simulink model "generic_Truck_And_Trailer"  (R2025a)
settings: Solver=VariableStepAuto  StartTime=0.0  StopTime=350  FixedStep=0.01  MaxStep=0.001  RelTol=1e-3  EnableMultiTasking=on
libraries: TruckMaker4SL x250, simulink x1
(part 2 of 11)

== system generic_Truck_And_Trailer/TruckMaker/IPG Vehicle/CarAndTrailer ==
  Sync_In : Inport
  VhclCtrl.Steering : Inport  Port=2
  Vhcl.Wheel.In : Inport  Port=3
  Vhcl.Misc : Inport  Port=4
  CarAndTrailerUpd : Subsystem
  Forces : Subsystem
  Ground : Ground
  Kinematics : Subsystem
  Kinetics : Subsystem
  Steering : Subsystem
  Terminator : Terminator
  Terminator1 : Terminator
  Trailer : Subsystem
  Sync_Out : Outport  VectorParamsAs1DForOutWhenUnconnected=off
  Brake.IF.In : Outport  Port=2  VectorParamsAs1DForOutWhenUnconnected=off
  wires:
  Trailer/16(Vhcl.Wheel.RR4) -> CarAndTrailerUpd/16(Vhcl.Wheel.RR4)
  Trailer/15(Vhcl.Wheel.RL4) -> CarAndTrailerUpd/15(Vhcl.Wheel.RL4)
  Trailer/14(Vhcl.Wheel.RR3) -> CarAndTrailerUpd/14(Vhcl.Wheel.RR3)
  Trailer/13(Vhcl.Wheel.RL3) -> CarAndTrailerUpd/13(Vhcl.Wheel.RL3)
  Ground/1 -> CarAndTrailerUpd/18(Vhcl.Fr1A)
  Trailer/17(Car.Hitch.FrcTrq) -> CarAndTrailerUpd/17(Car.Hitch.FrcTrq)
  Trailer/12(Vhcl.Wheel.FR2) -> CarAndTrailerUpd/12(Vhcl.Wheel.FR2)
  Trailer/11(Vhcl.Wheel.FL2) -> CarAndTrailerUpd/11(Vhcl.Wheel.FL2)
  Trailer/10(Vhcl.Wheel.RR2) -> CarAndTrailerUpd/10(Vhcl.Wheel.RR2)
  Trailer/9(Vhcl.Wheel.RL2) -> CarAndTrailerUpd/9(Vhcl.Wheel.RL2)
  Trailer/8(Vhcl.Wheel.RR) -> CarAndTrailerUpd/8(Vhcl.Wheel.RR)
  Trailer/7(Vhcl.Wheel.RL) -> CarAndTrailerUpd/7(Vhcl.Wheel.RL)
  Trailer/6(Vhcl.Wheel.FR) -> CarAndTrailerUpd/6(Vhcl.Wheel.FR)
  Trailer/5(Vhcl.Wheel.FL) -> CarAndTrailerUpd/5(Vhcl.Wheel.FL)
  Trailer/4(Vhcl.PoI) -> CarAndTrailerUpd/4(Vhcl.PoI)
  Trailer/3(Vhcl.Motion) -> CarAndTrailerUpd/3(Vhcl.Motion)
  Trailer/2(Vhcl.Steering) -> CarAndTrailerUpd/2(Vhcl.Steering)
  Trailer/1(Sync_Out) -> CarAndTrailerUpd/1(Sync_In)
  CarAndTrailerUpd/2(Brake.IF.In) -> Brake.IF.In/1
  CarAndTrailerUpd/1(Sync_Out) -> Sync_Out/1
  Vhcl.Misc/1 -> Terminator1/1
  Vhcl.Wheel.In/1 -> Terminator/1
  Kinetics/6(WheelCarrier.Misc) -> Trailer/6(WheelCarrier.Misc)
  Kinetics/5(Car.Trq_T2W) -> Trailer/5(Car.Trq_T2W)
  Steering/2(Steer.IF) -> Kinematics/2(Steer.IF)
  Kinetics/4(Car.Fr1) -> Trailer/4(Car.Fr1)
  Kinetics/3(Car.Hitch) -> Trailer/3(Car.Hitch)
  Kinetics/2(Trailer.Load) -> Trailer/2(Trailer.Load)
  VhclCtrl.Steering/1 -> Steering/2(VhclCtrl.Steering)
  Sync_In/1 -> Steering/1(Sync_In)
  Steering/1(Sync_Out) -> Kinematics/1(Sync_In)
  Kinetics/1(Sync_Out) -> Trailer/1(Sync_In)
  Kinematics/5(lBuf) -> Forces/5(lBuf)
  Forces/4(Car.Load) -> Kinetics/4(Car.Load)
  Forces/2(Car.Virtual) -> Kinetics/2(Car.Virtual)
  Kinematics/2(lSpring) -> Forces/2(lSpring)
  Kinematics/3(vDamp) -> Forces/3(vDamp)
  Forces/3(Car.Aero) -> Kinetics/3(Car.Aero)
  Forces/1(Sync_Out) -> Kinetics/1(Sync_In)
  Kinematics/1(Sync_Out) -> Forces/1(Sync_In)
  Kinematics/4(lStabi) -> Forces/4(lStabi)
  Kinematics/6(tWheelCarrier_z) -> Forces/6(tWheelCarrier_z)

== system generic_Truck_And_Trailer/TruckMaker/IPG Vehicle/PowerTrain ==
  note: When replacing the entire powertrain,
      | be sure to disable the IPG powertrain model by using the powertrain
      | model 'Model Manager off' in the vehicle GUI.
  note: <Your model here>
  Sync_In : Inport
  Vhcl.Wheel.PT : Inport  Port=2
  VhclCtrl.PT : Inport  Port=3
  BusCreator : BusCreator  Inputs=99
  Demux : Demux  Outputs=99
      settings: DisplayOption=none
  Gain : Gain
  PowerTrain : S-Function  FunctionName=TM_Sfun  Parameters='PowerTrain'  SFunctionDeploymentMode=off  EnableBusSupport=off
  PowerTrainUpd : S-Function  FunctionName=TM_Sfun  Parameters='PowerTrainUpd'  SFunctionDeploymentMode=off  EnableBusSupport=off
  Sum : Sum  Inputs=|++
  Sync_Out : Outport  VectorParamsAs1DForOutWhenUnconnected=off
  WRR_Trq-drive : Outport  Port=2
  wires:
  Demux/97 -> BusCreator/97  "PT IF WRR4 Trq_Supp2WC"
  Demux/95 -> BusCreator/95  "PT IF WRR4 Trq_B2W"
  Demux/92 -> BusCreator/92  "PT IF WRL4 Trq_BrakeReg_max"
  Demux/88 -> BusCreator/88  "PT IF WRL4 Trq_B2W"
  Demux/89 -> BusCreator/89  "PT IF WRL4 Trq_Drive"
  Demux/86 -> BusCreator/86  "PT IF WRL4 rot"
  Demux/91 -> BusCreator/91  "PT IF WRL4 Trq_BrakeReg"
  Demux/84 -> BusCreator/84  "PT IF WRR3 Trq_BrakeReg"
  Demux/83 -> BusCreator/83  "PT IF WRR3 Trq_Supp2WC"
  Demux/82 -> BusCreator/82  "PT IF WRR3 Trq_Drive"
  Demux/78 -> BusCreator/78  "PT IF WRL3 Trq_BrakeReg_max"
  Demux/87 -> BusCreator/87  "PT IF WRL4 rotv"
  Demux/77 -> BusCreator/77  "PT IF WRL3 Trq_BrakeReg"
  Demux/75 -> BusCreator/75  "PT IF WRL3 Trq_Drive"
  Demux/73 -> BusCreator/73  "PT IF WRL3 rotv"
  Demux/72 -> BusCreator/72  "PT IF WRL3 rot"
  Demux/71 -> BusCreator/71  "PT IF WFR2 Trq_BrakeReg_max"
  Demux/70 -> BusCreator/70  "PT IF WFR2 Trq_BrakeReg"
  Demux/67 -> BusCreator/67  "PT IF WFR2 Trq_B2W"
  Demux/66 -> BusCreator/66  "PT IF WFR2 rotv"
  Demux/80 -> BusCreator/80  "PT IF WRR3 rotv"
  Demux/65 -> BusCreator/65  "PT IF WFR2 rot"
  Demux/76 -> BusCreator/76  "PT IF WRL3 Trq_Supp2WC"
  Demux/63 -> BusCreator/63  "PT IF WFL2 Trq_BrakeReg"
  Demux/74 -> BusCreator/74  "PT IF WRL3 Trq_B2W"
  Demux/69 -> BusCreator/69  "PT IF WFR2 Trq_Supp2WC"
  Demux/58 -> BusCreator/58  "PT IF WFL2 rot"
  Demux/68 -> BusCreator/68  "PT IF WFR2 Trq_Drive"
  Demux/56 -> BusCreator/56  "PT IF WRR2 Trq_BrakeReg"
  Demux/61 -> BusCreator/61  "PT IF WFL2 Trq_Drive"
  Demux/24 -> BusCreator/24  "PT IF WFR rotv"
  BusCreator/1 -> PowerTrainUpd/2
  Demux/20 -> BusCreator/20  "PT IF WFL Trq_Supp2WC"
  Demux/13 -> BusCreator/13  "PT IF Trq_Supp2BdyEng x"
  Demux/99 -> BusCreator/99  "PT IF WRR4 Trq_BrakeReg_max"
  Demux/19 -> BusCreator/19  "PT IF WFL Trq_Drive"
  Demux/33 -> Sum/1, BusCreator/33  "PT IF WRL Trq_Drive"
  Demux/29 -> BusCreator/29  "PT IF WFR Trq_BrakeReg_max"
  Demux/64 -> BusCreator/64  "PT IF WFL2 Trq_BrakeReg_max"
  Demux/57 -> BusCreator/57  "PT IF WRR2 Trq_BrakeReg_max"
  Demux/42 -> BusCreator/42  "PT IF WRR Trq_BrakeReg"
  Demux/16 -> BusCreator/16  "PT IF WFL rot"
  Demux/26 -> BusCreator/26  "PT IF WFR Trq_Drive"
  PowerTrainUpd/1 -> Sync_Out/1
  Demux/93 -> BusCreator/93  "PT IF WRR4 rot"
  Demux/79 -> BusCreator/79  "PT IF WRR3 rot"
  Demux/37 -> BusCreator/37  "PT IF WRR rot"
  Demux/15 -> BusCreator/15  "PT IF DL_iDiff_mean"
  Demux/4 -> BusCreator/4  "PT IF OperationError"
  Demux/59 -> BusCreator/59  "PT IF WFL2 rotv"
  Demux/11 -> BusCreator/11  "PT IF Trq_Supp2Bdy1B y"
  Demux/90 -> BusCreator/90  "PT IF WRL4 Trq_Supp2WC"
  Demux/9 -> BusCreator/9  "PT IF Trq_Supp2Bdy1 z"
  Demux/1 -> BusCreator/1  "PT IF Ignition"
  Demux/98 -> BusCreator/98  "PT IF WRR4 Trq_BrakeReg"
  Demux/17 -> BusCreator/17  "PT IF WFL rotv"
  Sync_In/1 -> PowerTrain/1
  PowerTrain/2 -> Demux/1
  Vhcl.Wheel.PT/1 -> PowerTrain/2
  Demux/14 -> BusCreator/14  "PT IF Trq_Supp2BdyEng y"
  Demux/8 -> BusCreator/8  "PT IF Trq_Supp2Bdy1 y"
  PowerTrain/1 -> PowerTrainUpd/1  "Sync"
  Demux/40 -> Sum/2, BusCreator/40  "PT IF WRR Trq_Drive"
  Demux/12 -> BusCreator/12  "PT IF Trq_Supp2Bdy1B z"
  Demux/2 -> BusCreator/2  "PT IF SelectorCtrl"
  Demux/22 -> BusCreator/22  "PT IF WFL Trq_BrakeReg_max"
  Demux/3 -> BusCreator/3  "PT IF OperationState"
  Demux/10 -> BusCreator/10  "PT IF Trq_Supp2Bdy1B x"
  Demux/18 -> BusCreator/18  "PT IF WFL Trq_B2W"
  Demux/6 -> BusCreator/6  "PT IF Engine_rotv"
  Demux/5 -> BusCreator/5  "PT IF GearNo"
  Demux/27 -> BusCreator/27  "PT IF WFR Trq_Supp2WC"
  Demux/52 -> BusCreator/52  "PT IF WRR2 rotv"
  Demux/28 -> BusCreator/28  "PT IF WFR Trq_BrakeReg"
  Demux/41 -> BusCreator/41  "PT IF WRR Trq_Supp2WC"
  Demux/31 -> BusCreator/31  "PT IF WRL rotv"
  Demux/94 -> BusCreator/94  "PT IF WRR4 rotv"
  Demux/55 -> BusCreator/55  "PT IF WRR2 Trq_Supp2WC"
  Demux/32 -> BusCreator/32  "PT IF WRL Trq_B2W"
  Demux/35 -> BusCreator/35  "PT IF WRL Trq_BrakeReg"
  Demux/25 -> BusCreator/25  "PT IF WFR Trq_B2W"
  Demux/39 -> BusCreator/39  "PT IF WRR Trq_B2W"
  Demux/38 -> BusCreator/38  "PT IF WRR rotv"
  Demux/21 -> BusCreator/21  "PT IF WFL Trq_BrakeReg"
  VhclCtrl.PT/1 -> PowerTrain/3
  Demux/36 -> BusCreator/36  "PT IF WRL Trq_BrakeReg_max"
  Demux/60 -> BusCreator/60  "PT IF WFL2 Trq_B2W"
  Demux/43 -> BusCreator/43  "PT IF WRR Trq_BrakeReg_max"
  Demux/44 -> BusCreator/44  "PT IF WRL2 rot"
  Demux/81 -> BusCreator/81  "PT IF WRR3 Trq_B2W"
  Demux/30 -> BusCreator/30  "PT IF WRL rot"
  Demux/45 -> BusCreator/45  "PT IF WRL2 rotv"
  Demux/23 -> BusCreator/23  "PT IF WFR rot"
  Demux/46 -> BusCreator/46  "PT IF WRL2 Trq_B2W"
  Demux/96 -> BusCreator/96  "PT IF WRR4 Trq_Drive"
  Demux/54 -> BusCreator/54  "PT IF WRR2 Trq_Drive"
  Demux/85 -> BusCreator/85  "PT IF WRR3 Trq_BrakeReg_max"
  Demux/47 -> BusCreator/47  "PT IF WRL2 Trq_Drive"
  Demux/62 -> BusCreator/62  "PT IF WFL2 Trq_Supp2WC"
  Demux/7 -> BusCreator/7  "PT IF Trq_Supp2Bdy1 x"
  Demux/48 -> BusCreator/48  "PT IF WRL2 Trq_Supp2WC"
  Demux/34 -> BusCreator/34  "PT IF WRL Trq_Supp2WC"
  Demux/49 -> BusCreator/49  "PT IF WRL2 Trq_BrakeReg"
  Demux/50 -> BusCreator/50  "PT IF WRL2 Trq_BrakeReg_max"
  Demux/51 -> BusCreator/51  "PT IF WRR2 rot"
  Demux/53 -> BusCreator/53  "PT IF WRR2 Trq_B2W"
  Sum/1 -> Gain/1
  Gain/1 -> WRR_Trq-drive/1

== system generic_Truck_And_Trailer/TruckMaker/Subsystem1/Measurements from IMU ==
  Acc_x : TruckMaker4SL/Read CM Dict  xname=Sensor.Inertial.Vhcl.VchBdy.Acc_B.x  xsync=off  xstime=Continuous
      settings: SourceProductName=TruckMaker4SL
  Acc_x1 : TruckMaker4SL/Read CM Dict  xname=Vhcl.RL.rotv  xsync=off  xstime=Continuous
      settings: SourceProductName=TruckMaker4SL
  Acc_x2 : TruckMaker4SL/Read CM Dict  xname=Vhcl.RR.rotv  xsync=off  xstime=Continuous
      settings: SourceProductName=TruckMaker4SL
  Acc_x3 : TruckMaker4SL/Read CM Dict  xname=Tr.WheelSpd_ML  xsync=off  xstime=Continuous
      settings: SourceProductName=TruckMaker4SL
  Acc_x4 : TruckMaker4SL/Read CM Dict  xname=Tr.WheelSpd_MR  xsync=off  xstime=Continuous
      settings: SourceProductName=TruckMaker4SL
  Acc_y : TruckMaker4SL/Read CM Dict  xname=Sensor.Inertial.Vhcl.VchBdy.Acc_B.y  xsync=off  xstime=Continuous
      settings: SourceProductName=TruckMaker4SL
  FYh : TruckMaker4SL/Read CM Dict  xname=Tr.Hitch.Frc2Tr.y_1  xsync=off  xstime=Continuous
      settings: SourceProductName=TruckMaker4SL
  Gain : Gain
  Omega_z : TruckMaker4SL/Read CM Dict  xname=Sensor.Inertial.Vhcl.VchBdy.Omega_B.z  xsync=off  xstime=Continuous
      settings: SourceProductName=TruckMaker4SL
  Vel_x : TruckMaker4SL/Read CM Dict  xname=Sensor.Inertial.Vhcl.VchBdy.Vel_B.x  xsync=off  xstime=Continuous
      settings: SourceProductName=TruckMaker4SL
  Vel_y : TruckMaker4SL/Read CM Dict  xname=Sensor.Inertial.Vhcl.VchBdy.Vel_B.y  xsync=off  xstime=Continuous
      settings: SourceProductName=TruckMaker4SL
  acc_x : Outport
  acc_y : Outport  Port=2
  vel_x : Outport  Port=3
  vel_y : Outport  Port=4
  wz : Outport  Port=5
  omega_rl : Outport  Port=6
  omega_rr : Outport  Port=7
  omega_tr_ML : Outport  Port=8
  omega_tr_MR : Outport  Port=9
  FYH : Outport  Port=10
  wires:
  Omega_z/1 -> wz/1
  Vel_x/1 -> vel_x/1
  Vel_y/1 -> vel_y/1
  Acc_x/1 -> acc_x/1
  Acc_y/1 -> acc_y/1
  Acc_x2/1 -> omega_rr/1
  Acc_x1/1 -> omega_rl/1
  Acc_x3/1 -> omega_tr_ML/1
  Acc_x4/1 -> omega_tr_MR/1
  Gain/1 -> FYH/1
  FYh/1 -> Gain/1

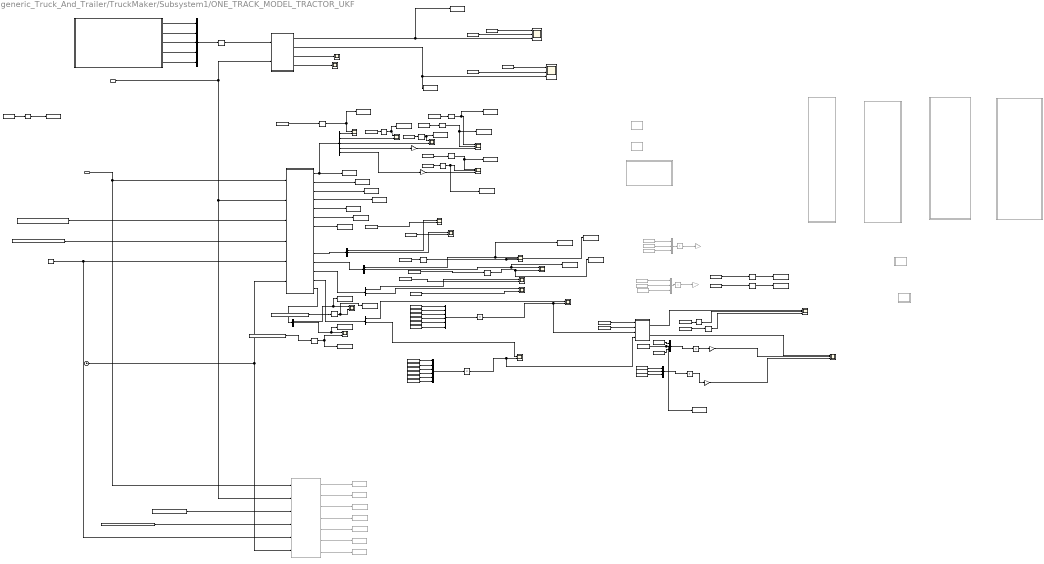
== system generic_Truck_And_Trailer/TruckMaker/Subsystem1/ONE_TRACK_MODEL_TRACTOR_UKF ==
  z : Inport
  u : Inport  Port=2
  "CF " : Scope  NumInputPorts=3
      settings: ActiveDisplayYMinimum=-12.263034323337607  ActiveDisplayYMaximum=-4.9489164501428942  DataLoggingVariableName=ScopeData23
  CF 1 : Scope  NumInputPorts=3
      settings: ActiveDisplayYMinimum=-10.797860186662938  ActiveDisplayYMaximum=-3.0037046797887497  DataLoggingVariableName=ScopeData30
  CR : Scope  NumInputPorts=3
      settings: ActiveDisplayYMinimum=-11.701585356235972  ActiveDisplayYMaximum=4.5045535239425494  DataLoggingVariableName=ScopeData24
  CR1 : Scope  NumInputPorts=3
      settings: ActiveDisplayYMinimum=-13.474282112558932  ActiveDisplayYMaximum=-8.0648262356989679  DataLoggingVariableName=ScopeData31
  CYRL : TruckMaker4SL/Read CM Dict  xname=CyRL  xsync=off  xstime=Continuous
      settings: SourceProductName=TruckMaker4SL
  CYRL1 : TruckMaker4SL/Read CM Dict  xname=CyRL  xsync=off  xstime=Continuous
      settings: SourceProductName=TruckMaker4SL
  CYRR : TruckMaker4SL/Read CM Dict  xname=CyRR  xsync=off  xstime=Continuous
      settings: SourceProductName=TruckMaker4SL
  CYRR1 : TruckMaker4SL/Read CM Dict  xname=CyRR  xsync=off  xstime=Continuous
      settings: SourceProductName=TruckMaker4SL
  CY_FL : TruckMaker4SL/Read CM Dict  xname=CyFL  xsync=off  xstime=Continuous
      settings: SourceProductName=TruckMaker4SL
  CY_FL1 : TruckMaker4SL/Read CM Dict  xname=CyFL  xsync=off  xstime=Continuous
      settings: SourceProductName=TruckMaker4SL
  CY_FR : TruckMaker4SL/Read CM Dict  xname=CyFR  xsync=off  xstime=Continuous
      settings: SourceProductName=TruckMaker4SL
  CY_FR1 : TruckMaker4SL/Read CM Dict  xname=CyFR  xsync=off  xstime=Continuous
      settings: SourceProductName=TruckMaker4SL
  Clock : Clock
  Constant : Constant  Value=0.01
  Demux : Demux  Outputs=5
  Demux1 : Demux  Outputs=3
  Demux2 : Demux  Outputs=3
  Demux3 : Demux  Outputs=2
  Demux4 : Demux  Outputs=2
  Demux5 : Demux  Outputs=3
  Fy_hitch : Scope  NumInputPorts=2
      settings: ActiveDisplayYMinimum=-39333.38762494702  ActiveDisplayYMaximum=91597.202407079487  DataLoggingVariableName=ScopeData48
  Fy_tire : Scope  NumInputPorts=2
      settings: ActiveDisplayYMinimum=-80059.601125398985  ActiveDisplayYMaximum=78399.9157079452  DataLoggingVariableName=ScopeData49
  Fz_hitch : Scope  NumInputPorts=2
      settings: ActiveDisplayYMinimum=23077.36897983135  ActiveDisplayYMaximum=152677.62430034793  DataLoggingVariableName=ScopeData47
  Fz_tire : Scope  NumInputPorts=2
      settings: ActiveDisplayYMinimum=23803.249495079042  ActiveDisplayYMaximum=292238.27856282709  DataLoggingVariableName=ScopeData50
  Gain : Gain  Gain=-1
  Gain1 : Gain  Gain=-1
  Gain2 : Gain  Gain=1/3
  Gain3 : Gain  Gain=1/3
  Gain4 : Gain  Commented=on  Gain=1/3
  Gain5 : Gain  Commented=on  Gain=1/3
  "Included_trailer " : MATLAB Function  Commented=on  TreatAsAtomicUnit=on
  Lateral_hastighet_hitch : Scope  NumInputPorts=2
      settings: ActiveDisplayYMinimum=-2.3776156180515082  ActiveDisplayYMaximum=2.859198442679677  DataLoggingVariableName=ScopeData44
  Lateral_hastighet_tire : Scope  NumInputPorts=2
      settings: ActiveDisplayYMinimum=-1.4861972675085433  ActiveDisplayYMaximum=1.1171708341440338  DataLoggingVariableName=ScopeData45
  Long_hastighet_hitch : Scope  NumInputPorts=2
      settings: ActiveDisplayYMinimum=17.114162676571183  ActiveDisplayYMaximum=17.332473790488748  DataLoggingVariableName=ScopeData43
  Long_hastighet_hitch_truck : Scope  NumInputPorts=2
      settings: ActiveDisplayYMinimum=16.981276621793427  ActiveDisplayYMaximum=17.35363637045576  DataLoggingVariableName=ScopeData52
  Long_hastighet_tire : Scope  NumInputPorts=2
      settings: ActiveDisplayYMinimum=-0.31075297440478167  ActiveDisplayYMaximum=26.970719906588407  DataLoggingVariableName=ScopeData46
  MATLAB Function : MATLAB Function  TreatAsAtomicUnit=on
  MATLAB Function1 : MATLAB Function  Commented=on  TreatAsAtomicUnit=on
  MATLAB Function2 : MATLAB Function  Commented=on  TreatAsAtomicUnit=on  SystemSampleTime=0.01
  MATLAB Function3 : MATLAB Function  TreatAsAtomicUnit=on
  Measurements from IMU : Subsystem  Description=Measurements from IMU Mounted in Vhcl position (3.6; 0.0;1.0)
  Mux : Mux  Inputs=6
  Mux1 : Mux  Inputs=6
  Mux2 : Mux  Inputs=5
  Mux3 : Mux  Inputs=3
  Mux4 : Mux  Inputs=3
  Mux5 : Mux  Commented=on  Inputs=3
  Mux6 : Mux  Commented=on  Inputs=3
  Q1 : Constant  Value="diag([2e-2 0.02 3e-3 0 0  0.02 1e-2 0.000 ]);"
  Q2 : Constant  Value="diag([5e-2 5e-2 3e-4 0 0  1e-3]);"
  R1 : Constant  Value=diag([2; 2; 0.6; 0.6; 0.005])/3;
  R3 : Constant  Value=diag([2; 2; 0.2; 0.2; 0.5; 0.5; 0.5; 0.5; 0.5; 5e4 ])/3;
  Read CM Dict : TruckMaker4SL/Read CM Dict  xname=Tr.YawVel  xsync=off  xstime=Continuous
      settings: SourceProductName=TruckMaker4SL
  Read CM Dict1 : TruckMaker4SL/Read CM Dict  xname=Sensor.Inertial.Tr.TR_IMU_hitch.Vel_B.x  xsync=off  xstime=Continuous
      settings: SourceProductName=TruckMaker4SL
  Read CM Dict10 : TruckMaker4SL/Read CM Dict  xname=Tr.CML.Tire.FrcC.y  xsync=off  xstime=Continuous
      settings: SourceProductName=TruckMaker4SL
  Read CM Dict11 : TruckMaker4SL/Read CM Dict  xname=Car.vy  xsync=off  xstime=Continuous
      settings: SourceProductName=TruckMaker4SL
  Read CM Dict12 : TruckMaker4SL/Read CM Dict  xname=Car.YawRate  xsync=off  xstime=Continuous
      settings: SourceProductName=TruckMaker4SL
  Read CM Dict13 : TruckMaker4SL/Read CM Dict  xname=Tr.CFR.Tire.FrcC.z  xsync=off  xstime=Continuous
      settings: SourceProductName=TruckMaker4SL
  Read CM Dict14 : TruckMaker4SL/Read CM Dict  xname=Tr.CML.Tire.FrcC.z  xsync=off  xstime=Continuous
      settings: SourceProductName=TruckMaker4SL
  Read CM Dict15 : TruckMaker4SL/Read CM Dict  xname=Tr.CMR.Tire.FrcC.z  xsync=off  xstime=Continuous
      settings: SourceProductName=TruckMaker4SL
  Read CM Dict16 : TruckMaker4SL/Read CM Dict  xname=Tr.CRL.Tire.FrcC.z  xsync=off  xstime=Continuous
      settings: SourceProductName=TruckMaker4SL
  Read CM Dict17 : TruckMaker4SL/Read CM Dict  xname=Tr.CRR.Tire.FrcC.z  xsync=off  xstime=Continuous
      settings: SourceProductName=TruckMaker4SL
  Read CM Dict18 : TruckMaker4SL/Read CM Dict  xname=Tr.CMR.Tire.FrcC.y  xsync=off  xstime=Continuous
      settings: SourceProductName=TruckMaker4SL
  Read CM Dict19 : TruckMaker4SL/Read CM Dict  xname=Tr.CRL.Tire.FrcC.y  xsync=off  xstime=Continuous
      settings: SourceProductName=TruckMaker4SL
  Read CM Dict2 : TruckMaker4SL/Read CM Dict  xname=Sensor.Inertial.Tr.TR_IMU_hitch.Vel_B.y  xsync=off  xstime=Continuous
      settings: SourceProductName=TruckMaker4SL
  Read CM Dict20 : TruckMaker4SL/Read CM Dict  xname=Tr.CRR.Tire.FrcC.y  xsync=off  xstime=Continuous
      settings: SourceProductName=TruckMaker4SL
  Read CM Dict21 : TruckMaker4SL/Read CM Dict  xname=Tr.CFL.Tire.FrcC.y  xsync=off  xstime=Continuous
      settings: SourceProductName=TruckMaker4SL
  Read CM Dict22 : TruckMaker4SL/Read CM Dict  xname=Sensor.Inertial.Tr.TR_IMU_Tire.Vel_B.x  xsync=off  xstime=Continuous
      settings: SourceProductName=TruckMaker4SL
  Read CM Dict23 : TruckMaker4SL/Read CM Dict  xname=Sensor.Inertial.Tr.TR_IMU_Tire.Vel_B.y  xsync=off  xstime=Continuous
      settings: SourceProductName=TruckMaker4SL
  Read CM Dict24 : TruckMaker4SL/Read CM Dict  xname=Tr.SlipAngleML  xsync=off  xstime=Continuous
      settings: SourceProductName=TruckMaker4SL
  Read CM Dict25 : TruckMaker4SL/Read CM Dict  xname=CyML_TR  xsync=off  xstime=Continuous
      settings: SourceProductName=TruckMaker4SL
  Read CM Dict26 : TruckMaker4SL/Read CM Dict  xname=CyMR_TR  xsync=off  xstime=Continuous
      settings: SourceProductName=TruckMaker4SL
  Read CM Dict27 : TruckMaker4SL/Read CM Dict  xname=Tr.SlipAngleFR  xsync=off  xstime=Continuous
      settings: SourceProductName=TruckMaker4SL
  Read CM Dict28 : TruckMaker4SL/Read CM Dict  xname=Tr.SlipAngleFL  xsync=off  xstime=Continuous
      settings: SourceProductName=TruckMaker4SL
  Read CM Dict29 : TruckMaker4SL/Read CM Dict  xname=Tr.SlipAngleRL  xsync=off  xstime=Continuous
      settings: SourceProductName=TruckMaker4SL
  Read CM Dict3 : TruckMaker4SL/Read CM Dict  xname=Sensor.Inertial.Tr.TR_IMU_Tire.Vel_B.x  xsync=off  xstime=Continuous
      settings: SourceProductName=TruckMaker4SL
  Read CM Dict30 : TruckMaker4SL/Read CM Dict  xname=Tr.SlipAngleMR  xsync=off  xstime=Continuous
      settings: SourceProductName=TruckMaker4SL
  Read CM Dict31 : TruckMaker4SL/Read CM Dict  xname=Tr.SlipAngleRR  xsync=off  xstime=Continuous
      settings: SourceProductName=TruckMaker4SL
  Read CM Dict32 : TruckMaker4SL/Read CM Dict  xname=Sensor.Inertial.Vhcl.Car_IMU_Hitch.Vel_B.x  xsync=off  xstime=Continuous
      settings: SourceProductName=TruckMaker4SL
  Read CM Dict33 : TruckMaker4SL/Read CM Dict  xname=Sensor.Inertial.Vhcl.Car_IMU_Hitch.Vel_B.y  xsync=off  xstime=Continuous
      settings: SourceProductName=TruckMaker4SL
  Read CM Dict34 : TruckMaker4SL/Read CM Dict  Commented=on  xname=CyFL_TR  xsync=off  xstime=Continuous
      settings: SourceProductName=TruckMaker4SL
  Read CM Dict35 : TruckMaker4SL/Read CM Dict  Commented=on  xname=CyFR_TR  xsync=off  xstime=Continuous
      settings: SourceProductName=TruckMaker4SL
  Read CM Dict36 : TruckMaker4SL/Read CM Dict  Commented=on  xname=CyML_TR  xsync=off  xstime=Continuous
      settings: SourceProductName=TruckMaker4SL
  Read CM Dict37 : TruckMaker4SL/Read CM Dict  Commented=on  xname=CyRL_TR  xsync=off  xstime=Continuous
      settings: SourceProductName=TruckMaker4SL
  Read CM Dict38 : TruckMaker4SL/Read CM Dict  Commented=on  xname=CyMR_TR  xsync=off  xstime=Continuous
      settings: SourceProductName=TruckMaker4SL
  Read CM Dict39 : TruckMaker4SL/Read CM Dict  Commented=on  xname=CyRR_TR  xsync=off  xstime=Continuous
      settings: SourceProductName=TruckMaker4SL
  Read CM Dict4 : TruckMaker4SL/Read CM Dict  xname=Sensor.Inertial.Tr.TR_IMU_Tire.Vel_B.y  xsync=off  xstime=Continuous
      settings: SourceProductName=TruckMaker4SL
  Read CM Dict40 : TruckMaker4SL/Read CM Dict  xname=CyMR_TR  xsync=off  xstime=Continuous
      settings: SourceProductName=TruckMaker4SL
  Read CM Dict41 : TruckMaker4SL/Read CM Dict  xname=CyML_TR  xsync=off  xstime=Continuous
      settings: SourceProductName=TruckMaker4SL
  Read CM Dict5 : TruckMaker4SL/Read CM Dict  xname=Tr.Hitch.Frc2Tr.y_1  xsync=off  xstime=Continuous
      settings: SourceProductName=TruckMaker4SL
  Read CM Dict6 : TruckMaker4SL/Read CM Dict  xname=Car.vx  xsync=off  xstime=Continuous
      settings: SourceProductName=TruckMaker4SL
  Read CM Dict7 : TruckMaker4SL/Read CM Dict  xname=Tr.Hitch.Frc2Tr.z_1  xsync=off  xstime=Continuous
      settings: SourceProductName=TruckMaker4SL
  Read CM Dict8 : TruckMaker4SL/Read CM Dict  xname=Tr.CFR.Tire.FrcC.y  xsync=off  xstime=Continuous
      settings: SourceProductName=TruckMaker4SL
  Read CM Dict9 : TruckMaker4SL/Read CM Dict  xname=Tr.CFL.Tire.FrcC.z  xsync=off  xstime=Continuous
      settings: SourceProductName=TruckMaker4SL
  SSA_F : Scope
      settings: ActiveDisplayYMinimum=-0.046315426334515186  ActiveDisplayYMaximum=0.00321973029301955  DataLoggingVariableName=ScopeData25
  SSA_R : Scope
      settings: ActiveDisplayYMinimum=19.809904868748255  ActiveDisplayYMaximum=19.861105266179973  DataLoggingVariableName=ScopeData26
  SideSlipAngle(SSA) : Scope  NumInputPorts=3
      settings: ActiveDisplayYMinimum=-0.058563230672732614  ActiveDisplayYMaximum=-0.0070357098526823911  DataLoggingVariableName=ScopeData51
  Sum of Elements{,1..3} (4 alike) : Sum  Inputs=+
  Sum of Elements4 : Sum  Commented=on  Inputs=+
  Sum of Elements5 : Sum  Commented=on  Inputs=+
  "TEST_Algorithm " : MATLAB Function  Commented=on  TreatAsAtomicUnit=on
  TSC_Ren_IPG_DATA : Scope  NumInputPorts=3
      settings: ActiveDisplayYMinimum=-10.986627521173382  ActiveDisplayYMaximum=-3.5607522765873121  DataLoggingVariableName=ScopeData42
  To Workspace : ToWorkspace  VariableName=P_sim  SaveFormat=Timeseries  SampleTime=-1
  To Workspace1 : ToWorkspace  VariableName=xhat_sim  SaveFormat=Timeseries  SampleTime=-1
  To Workspace10 : ToWorkspace  VariableName=CF_sim  SaveFormat=Timeseries  SampleTime=-1
  To Workspace11 : ToWorkspace  VariableName=dxdt_sim  SaveFormat=Timeseries  SampleTime=-1
  To Workspace12 : ToWorkspace  VariableName=innovation_sim  SaveFormat=Timeseries  SampleTime=-1
  To Workspace13 : ToWorkspace  VariableName=K_sim  SaveFormat=Timeseries  SampleTime=-1
  To Workspace14 : ToWorkspace  VariableName=S_sim  SaveFormat=Timeseries  SampleTime=-1
  To Workspace15 : ToWorkspace  VariableName=Z_pred_sim  SaveFormat=Timeseries  SampleTime=-1
  To Workspace16 : ToWorkspace  Commented=on  VariableName=P_sim1  SaveFormat=Timeseries  SampleTime=-1
  To Workspace17 : ToWorkspace  Commented=on  VariableName=xhat_sim1  SaveFormat=Timeseries  SampleTime=-1
  To Workspace18 : ToWorkspace  Commented=on  VariableName=dxdt_sim1  SaveFormat=Timeseries  SampleTime=-1
  To Workspace19 : ToWorkspace  Commented=on  VariableName=innovation_sim1  SaveFormat=Timeseries  SampleTime=-1
  To Workspace2 : ToWorkspace  VariableName=Car_vx  SaveFormat=Timeseries  SampleTime=-1
  To Workspace20 : ToWorkspace  Commented=on  VariableName=K_sim1  SaveFormat=Timeseries  SampleTime=-1
  To Workspace21 : ToWorkspace  Commented=on  VariableName=S_sim1  SaveFormat=Timeseries  SampleTime=-1
  To Workspace22 : ToWorkspace  Commented=on  VariableName=Z_pred_sim1  SaveFormat=Timeseries  SampleTime=-1
  To Workspace23 : ToWorkspace  VariableName=Tr_YawRate  SaveFormat=Timeseries  SampleTime=-1
  To Workspace24 : ToWorkspace  VariableName=Long_V_H_TK_estimate  SaveFormat=Timeseries  SampleTime=-1
  To Workspace25 : ToWorkspace  VariableName=Long_V_H_TK_Sen  SaveFormat=Timeseries  SampleTime=-1
  To Workspace26 : ToWorkspace  VariableName=Lat_V_H_TK_estimate  SaveFormat=Timeseries  SampleTime=-1
  To Workspace27 : ToWorkspace  VariableName=Lat_V_H_TK_Sen  SaveFormat=Timeseries  SampleTime=-1
  To Workspace28 : ToWorkspace  VariableName=Lat_V_H_TR_estimate  SaveFormat=Timeseries  SampleTime=-1
  To Workspace29 : ToWorkspace  VariableName=Lat_V_H_TR_Sen  SaveFormat=Timeseries  SampleTime=-1
  To Workspace3 : ToWorkspace  VariableName=Car_vy  SaveFormat=Timeseries  SampleTime=-1
  To Workspace30 : ToWorkspace  VariableName=Long_V_H_TR_estimate  SaveFormat=Timeseries  SampleTime=-1
  To Workspace31 : ToWorkspace  VariableName=Long_V_H_TR_Sen  SaveFormat=Timeseries  SampleTime=-1
  To Workspace32 : ToWorkspace  VariableName=CyML  SaveFormat=Timeseries  SampleTime=-1
  To Workspace33 : ToWorkspace  VariableName=CyMR  SaveFormat=Timeseries  SampleTime=-1
  To Workspace34 : ToWorkspace  VariableName=simout  SaveFormat=Timeseries  SampleTime=-1
  To Workspace4 : ToWorkspace  VariableName=Car_wz  SaveFormat=Timeseries  SampleTime=-1
  To Workspace5 : ToWorkspace  VariableName=CyFL  SaveFormat=Timeseries  SampleTime=-1
  To Workspace6 : ToWorkspace  VariableName=CyFR  SaveFormat=Timeseries  SampleTime=-1
  To Workspace7 : ToWorkspace  VariableName=CyRL  SaveFormat=Timeseries  SampleTime=-1
  To Workspace8 : ToWorkspace  VariableName=CyRR  SaveFormat=Timeseries  SampleTime=-1
  To Workspace9 : ToWorkspace  VariableName=CR_sim  SaveFormat=Timeseries  SampleTime=-1
  UKF_ONE_TRACK2 : MATLAB Function  Commented=on  TreatAsAtomicUnit=on  SystemSampleTime=0.01
  UKF_ONE_TRACK3 : MATLAB Function  Commented=on  TreatAsAtomicUnit=on  SystemSampleTime=0.01
  UKF_ONE_TRACK4 : MATLAB Function  Commented=on  TreatAsAtomicUnit=on  SystemSampleTime=0.01
  "UKF_ONE_TRACK_TRUCK_AND_TRAILER_WORKING_MODEL " : MATLAB Function  Commented=on  TreatAsAtomicUnit=on  SystemSampleTime=0.01
  UKF_ONE_TRACK_TruckAndTrailer : MATLAB Function  TreatAsAtomicUnit=on  SystemSampleTime=0.01
  "Working Model with 5 measurements " : MATLAB Function  Commented=on  TreatAsAtomicUnit=on
  Working Model with 7 measurements : MATLAB Function  Commented=on  TreatAsAtomicUnit=on
  Zero-Order Hold{,1..16} (17 alike) : ZeroOrderHold  SampleTime=0.01
  lateral_hastighet_hitch_truck : Scope  NumInputPorts=2
      settings: ActiveDisplayYMinimum=-1.3295004363082232  ActiveDisplayYMaximum=0.272932480462097  DataLoggingVariableName=ScopeData53
  vx : Scope  NumInputPorts=2
      settings: ActiveDisplayYMinimum=15.532965030483135  ActiveDisplayYMaximum=19.510688761225374  DataLoggingVariableName=ScopeData34
  vy : Scope  NumInputPorts=2
      settings: ActiveDisplayYMinimum=-0.016234882238860611  ActiveDisplayYMaximum=0.084455127817541567  DataLoggingVariableName=ScopeData35
  wz : Scope  NumInputPorts=2
      settings: ActiveDisplayYMinimum=-0.21237399330212148  ActiveDisplayYMaximum=0.50990512712526215  DataLoggingVariableName=ScopeData36
  wires:
  MATLAB Function/1(Cf) -> To Workspace10/1, "CF "/3  "Cmptd_Cf"
  Read CM Dict6/1 -> Zero-Order Hold1/1
  CY_FR1/1 -> Zero-Order Hold4/1  "CyFR"
  Demux/1 -> vx/2  "est_vx"
  UKF_ONE_TRACK_TruckAndTrailer/2(P) -> To Workspace/1
  UKF_ONE_TRACK_TruckAndTrailer/1(xhat) -> Demux/1, To Workspace1/1  "State_estimates"
  R3/1 -> UKF_ONE_TRACK_TruckAndTrailer/4(R)
  CYRL1/1 -> Zero-Order Hold6/1  "CyRL"
  Gain/1 -> CR1/3  "est_CR"
  CYRL/1 -> CR/1  "CyRL"
  Constant/1 -> MATLAB Function2/5(Ts), UKF_ONE_TRACK_TruckAndTrailer/5(Ts)
  Read CM Dict12/1 -> Zero-Order Hold3/1
  MATLAB Function/4(alpha_r) -> SSA_R/1
  CYRR1/1 -> Zero-Order Hold7/1  "CyRR"
  CYRR/1 -> CR/2  "CyRR"
  Demux/2 -> vy/2  "est_vy"
  MATLAB Function/2(Cr) -> To Workspace9/1, CR/3  "cmptd_R"
  CY_FL1/1 -> Zero-Order Hold5/1  "CyFL"
  Read CM Dict11/1 -> Zero-Order Hold2/1
  Demux/5 -> Gain/1  "cmptd_R"
  CY_FL/1 -> "CF "/1  "CyFL"
  Demux/3 -> wz/2  "est_wz"
  CY_FR/1 -> "CF "/2  "CyFR"
  MATLAB Function/3(alpha_f) -> SSA_F/1
  Demux/4 -> Gain1/1  "Cmptd_Cf"
  Gain1/1 -> CF 1/3  "Est_CF"
  UKF_ONE_TRACK_TruckAndTrailer/3(dxdt) -> To Workspace11/1
  Q1/1 -> UKF_ONE_TRACK_TruckAndTrailer/3(Q)
  u/1 -> MATLAB Function/2(u), MATLAB Function2/2(u), UKF_ONE_TRACK_TruckAndTrailer/2(u)
  UKF_ONE_TRACK_TruckAndTrailer/4(innovation) -> To Workspace12/1
  UKF_ONE_TRACK_TruckAndTrailer/5(K_out) -> To Workspace13/1
  UKF_ONE_TRACK_TruckAndTrailer/6(S_out) -> To Workspace14/1
  UKF_ONE_TRACK_TruckAndTrailer/7(z_pred_out) -> To Workspace15/1
  z/1 -> MATLAB Function2/1(z), UKF_ONE_TRACK_TruckAndTrailer/1(z)
  Measurements from IMU/1(acc_x) -> Mux2/1
  Measurements from IMU/4(vel_y) -> Mux2/4
  Measurements from IMU/3(vel_x) -> Mux2/3
  Mux2/1 -> Zero-Order Hold/1
  Measurements from IMU/2(acc_y) -> Mux2/2
  Measurements from IMU/5(wz) -> Mux2/5
  Clock/1 -> UKF_ONE_TRACK_TruckAndTrailer/6(data), MATLAB Function2/6(data)
  MATLAB Function2/7(z_pred_out) -> To Workspace22/1
  MATLAB Function2/6(S_out) -> To Workspace21/1
  MATLAB Function2/5(K_out) -> To Workspace20/1
  MATLAB Function2/4(innovation) -> To Workspace19/1
  MATLAB Function2/3(dxdt) -> To Workspace18/1
  MATLAB Function2/1(xhat) -> To Workspace17/1  "State_estimates"
  MATLAB Function2/2(P) -> To Workspace16/1
  R1/1 -> MATLAB Function2/4(R)
  Q2/1 -> MATLAB Function2/3(Q)
  Zero-Order Hold/1 -> MATLAB Function/1(z)
  Zero-Order Hold1/1 -> To Workspace2/1, vx/1
  Zero-Order Hold2/1 -> To Workspace3/1, vy/1
  Zero-Order Hold3/1 -> To Workspace4/1, wz/1
  Zero-Order Hold4/1 -> To Workspace6/1, CF 1/2
  Zero-Order Hold5/1 -> To Workspace5/1, CF 1/1
  Zero-Order Hold6/1 -> To Workspace7/1, CR1/1
  Zero-Order Hold7/1 -> To Workspace8/1, CR1/2
  Read CM Dict/1 -> Zero-Order Hold8/1
  Zero-Order Hold8/1 -> To Workspace23/1
  UKF_ONE_TRACK_TruckAndTrailer/10(trailer_v_hitch) -> Demux1/1  "Estimated_V_hitch_trailer"
  Demux1/1 -> Long_hastighet_hitch/1  "Long_Hitch_Velocity_trailer_Estimated"
  Read CM Dict1/1 -> Long_hastighet_hitch/2  "Long_Hitch_Velocity_trailer_Sensor"
  Read CM Dict2/1 -> Lateral_hastighet_hitch/2  "Lateral_Hitch_Velocity_trailer_Sensor"
  Demux1/2 -> Lateral_hastighet_hitch/1  "Lateral_Hitch_Velocity_trailer_Estimated"
  Read CM Dict4/1 -> Zero-Order Hold11/1  "Lateral_tire_Velocity_trailer_Sensor"
  UKF_ONE_TRACK_TruckAndTrailer/11(trailer_v_axle) -> Demux2/1  "Estimated_V_tire_trailer"
  UKF_ONE_TRACK_TruckAndTrailer/12(trailer_F_hitch) -> Demux3/1  "F_hitch_trailer_Estimated"
  Demux3/1 -> Fy_hitch/1  "Fy_hitch_trailer_estmated"
  Read CM Dict5/1 -> Fy_hitch/2  "Fy_hitch_trailer_IPG"
  Read CM Dict7/1 -> Fz_hitch/2  "Fz_hitch_trailer_IPG"
  Demux3/2 -> Fz_hitch/1  "Fz_hitch_trailer_estmated"
  Demux4/2 -> Fz_tire/1  "Fz_CP/tire_trailer_estmated"
  Sum of Elements/1 -> MATLAB Function3/4(Fz_tire), Fz_tire/2  "Fz_tire_trailer_IPG"
  Demux4/1 -> Fy_tire/1  "Fy_CP/tire_trailer_estmated"
  UKF_ONE_TRACK_TruckAndTrailer/13(trailer_F_tire) -> Demux4/1  "F_tire/contactpatch_trailer_Estimated"
  Sum of Elements1/1 -> MATLAB Function3/3(Fy_tire), Fy_tire/2  "Fy_tire_trailer_IPG"
  Read CM Dict9/1 -> Mux/1  "Fz_tire_trailer_IPG"
  Read CM Dict13/1 -> Mux/2  "Fz_tire_trailer_IPG"
  Read CM Dict14/1 -> Mux/3  "Fz_tire_trailer_IPG"
  Read CM Dict15/1 -> Mux/4  "Fz_tire_trailer_IPG"
  Read CM Dict16/1 -> Mux/5  "Fz_tire_trailer_IPG"
  Read CM Dict17/1 -> Mux/6  "Fz_tire_trailer_IPG"
  Mux/1 -> Sum of Elements/1
  Mux1/1 -> Sum of Elements1/1
  Read CM Dict21/1 -> Mux1/1  "Fy_tire_trailer_IPG"
  Read CM Dict8/1 -> Mux1/2  "Fy_tire_trailer_IPG"
  Read CM Dict10/1 -> Mux1/3  "Fy_tire_trailer_IPG"
  Read CM Dict18/1 -> Mux1/4  "Fy_tire_trailer_IPG"
  Read CM Dict19/1 -> Mux1/5  "Fy_tire_trailer_IPG"
  Read CM Dict20/1 -> Mux1/6  "Fy_tire_trailer_IPG"
  Read CM Dict22/1 -> MATLAB Function3/1(vx_tire)  "Long_tire_Velocity_trailer_Sensor"
  Read CM Dict23/1 -> MATLAB Function3/2(vy_tire)  "Lateral_tire_Velocity_trailer_Sensor"
  MATLAB Function3/1(TCS_trailer) -> TSC_Ren_IPG_DATA/1
  MATLAB Function3/2(SSA) -> SideSlipAngle(SSA)/1  "SideSlipAngle_computed"
  Gain2/1 -> SideSlipAngle(SSA)/2  "IPG_SideSLipAngle"
  Read CM Dict25/1 -> Zero-Order Hold13/1  "IPG_CyML"
  Read CM Dict26/1 -> Zero-Order Hold14/1  "IPG_CyMR"
  Read CM Dict27/1 -> Mux4/1  "IPG_SideSLipAngle"
  Sum of Elements2/1 -> Gain2/1
  Read CM Dict28/1 -> Mux3/3  "IPG_SideSLipAngle"
  Read CM Dict24/1 -> To Workspace34/1, Mux3/2  "IPG_SideSLipAngle"
  Read CM Dict29/1 -> Mux3/1  "IPG_SideSLipAngle"
  Mux3/1 -> Sum of Elements2/1
  Gain3/1 -> SideSlipAngle(SSA)/3  "IPG_SideSLipAngle"
  Mux4/1 -> Sum of Elements3/1
  Sum of Elements3/1 -> Gain3/1
  Read CM Dict30/1 -> Mux4/2  "IPG_SideSLipAngle"
  Read CM Dict31/1 -> Mux4/3  "IPG_SideSLipAngle"
  UKF_ONE_TRACK_TruckAndTrailer/14(truck_v_hitch) -> Demux5/1  "truck_hastighet_Hitch"
  Demux5/1 -> Long_hastighet_hitch_truck/1, To Workspace24/1  "Long_hastighet_hitch_truck_estimatet"
  Read CM Dict32/1 -> Zero-Order Hold9/1  "Long_Hitch_Velocity_trailer_Sensor"
  Read CM Dict33/1 -> Zero-Order Hold10/1  "Long_Hitch_Velocity_trailer_Sensor"
  Demux5/2 -> lateral_hastighet_hitch_truck/1, To Workspace26/1  "Lat_hastighet_hitch_truck_estimate"
  Demux2/2 -> To Workspace28/1, Lateral_hastighet_tire/1  "Lat_hastighet_tire_truck_estimate"
  Demux2/1 -> To Workspace30/1, Long_hastighet_tire/1  "Lat_hastighet_hitch_trailer_estimate"
  Read CM Dict3/1 -> Zero-Order Hold12/1  "Lateral_tire_Velocity_trailer_Sensor"
  Zero-Order Hold9/1 -> Long_hastighet_hitch_truck/2, To Workspace25/1
  Zero-Order Hold10/1 -> lateral_hastighet_hitch_truck/2, To Workspace27/1
  Zero-Order Hold11/1 -> Lateral_hastighet_tire/2, To Workspace29/1
  Zero-Order Hold12/1 -> To Workspace31/1, Long_hastighet_tire/2
  Zero-Order Hold13/1 -> TSC_Ren_IPG_DATA/2
  Zero-Order Hold14/1 -> TSC_Ren_IPG_DATA/3
  Zero-Order Hold15/1 -> To Workspace32/1
  Read CM Dict35/1 -> Mux5/1  "IPG_CyMR"
  Read CM Dict34/1 -> Mux6/1  "IPG_CyML"
  Zero-Order Hold16/1 -> To Workspace33/1
  Read CM Dict36/1 -> Mux6/2  "IPG_CyML"
  Read CM Dict37/1 -> Mux6/3  "IPG_CyML"
  Mux6/1 -> Sum of Elements4/1
  Read CM Dict38/1 -> Mux5/2  "IPG_CyMR"
  Read CM Dict39/1 -> Mux5/3  "IPG_CyMR"
  Sum of Elements4/1 -> Gain4/1
  Sum of Elements5/1 -> Gain5/1
  Mux5/1 -> Sum of Elements5/1
  Read CM Dict40/1 -> Zero-Order Hold16/1  "IPG_CyMR"
  Read CM Dict41/1 -> Zero-Order Hold15/1  "IPG_CyML"

== system generic_Truck_And_Trailer/TruckMaker/Subsystem1/Subsystem ==
  Ackerman Angle : Subsystem  Commented=on
  Average Steering Angle : Subsystem
  Bromsmoment  trailer rear : Subsystem
  "Bromsmoment fram " : Subsystem
  Bromsmoment rear 1 : Subsystem
  FXh : TruckMaker4SL/Read CM Dict  xname=Tr.Hitch.Frc2Tr.x_1  xsync=off  xstime=Continuous
      settings: SourceProductName=TruckMaker4SL
  Minus : Sum  Inputs=+-
  Read CM Dict : TruckMaker4SL/Read CM Dict  xname=Tr.Yaw  xsync=off  xstime=Continuous
      settings: SourceProductName=TruckMaker4SL
  Read CM Dict1 : TruckMaker4SL/Read CM Dict  xname=Car.Yaw  xsync=off  xstime=Continuous
      settings: SourceProductName=TruckMaker4SL
  Scope : Scope
      settings: DataLoggingVariableName=ScopeData39
  Scope1 : Scope
      settings: ActiveDisplayYMinimum=-1813.6997625686197  ActiveDisplayYMaximum=16323.297863117581  DataLoggingVariableName=ScopeData40
  Scope2 : Scope
      settings: ActiveDisplayYMinimum=-1  ActiveDisplayYMaximum=1  DataLoggingVariableName=ScopeData41
  To Workspace : ToWorkspace  VariableName=psi  SaveFormat=Timeseries  SampleTime=-1
  Trq_RL : TruckMaker4SL/Read CM Dict  xname=Vhcl.RL.Trq_Drive  xsync=off  xstime=Continuous
      settings: SourceProductName=TruckMaker4SL
  Trq_RR : TruckMaker4SL/Read CM Dict  xname=Vhcl.RR.Trq_Drive  xsync=off  xstime=Continuous
      settings: SourceProductName=TruckMaker4SL
  Zero-Order Hold2 : ZeroOrderHold  SampleTime=0.01
  "Average_steering " : Outport
  Trq_T2W_RL : Outport  Port=2
  Trq_T2W_RR : Outport  Port=3
  FXH : Outport  Port=4
  TBF : Outport  Port=5
  TBR : Outport  Port=6
  TBR_Tr : Outport  Port=7
  wires:
  Trq_RL/1 -> Trq_T2W_RL/1
  Trq_RR/1 -> Trq_T2W_RR/1
  Average Steering Angle/1("Average_steering ") -> "Average_steering "/1
  FXh/1 -> FXH/1
  Bromsmoment rear 1/1("Average_Bromsmomet ") -> Scope2/1, TBR/1
  Bromsmoment  trailer rear/1("Average_Bromsmomet ") -> Scope/1, TBR_Tr/1
  Read CM Dict/1 -> Minus/1
  Read CM Dict1/1 -> Minus/2
  Minus/1 -> Zero-Order Hold2/1
  "Bromsmoment fram "/1("Average_Bromsmomet ") -> Scope1/1, TBF/1
  Zero-Order Hold2/1 -> To Workspace/1

== system generic_Truck_And_Trailer/TruckMaker/Subsystem1/Subsystem_Noisey Measurements ==
  Acc_x : TruckMaker4SL/Read CM Dict  xname=Vhcl.RL.rotv  xsync=off  xstime=Continuous
      settings: SourceProductName=TruckMaker4SL
  Acc_x1 : TruckMaker4SL/Read CM Dict  xname=Vhcl.RR.rotv  xsync=off  xstime=Continuous
      settings: SourceProductName=TruckMaker4SL
  Acc_x3 : TruckMaker4SL/Read CM Dict  xname=Tr.WheelSpd_FL  xsync=off  xstime=Continuous
      settings: SourceProductName=TruckMaker4SL
  Acc_x4 : TruckMaker4SL/Read CM Dict  xname=Tr.WheelSpd_FR  xsync=off  xstime=Continuous
      settings: SourceProductName=TruckMaker4SL
  Demux : Demux  Outputs=2
  Demux1 : Demux  Outputs=2
  Demux2 : Demux  Outputs=2
  Demux3 : Demux  Outputs=1
  FYh : TruckMaker4SL/Read CM Dict  xname=Tr.Hitch.Frc2Tr.y_1  xsync=off  xstime=Continuous
      settings: SourceProductName=TruckMaker4SL
  Gain : Gain
  MATLAB Function : MATLAB Function  TreatAsAtomicUnit=on
  MATLAB Function1 : MATLAB Function  TreatAsAtomicUnit=on
  MATLAB Function2 : MATLAB Function  TreatAsAtomicUnit=on
  MATLAB Function3 : MATLAB Function  TreatAsAtomicUnit=on
  MATLAB Function5 : MATLAB Function  TreatAsAtomicUnit=on
  Measurements from IMU : Subsystem  Description=Measurements from IMU Mounted in Vhcl position (3.6; 0.0;1.0)
  Mux : Mux  Inputs=3
  Mux1 : Mux  Inputs=3
  Mux2 : Mux  Inputs=6
  Mux3 : Mux  Inputs=3
  Mux5 : Mux  Inputs=2
  Mux6 : Mux  Inputs=2
  Scope : Scope
      settings: ActiveDisplayYMinimum=-5.6580655588196418  ActiveDisplayYMaximum=20.488387754127984  DataLoggingVariableName=ScopeData37
  Out1 : Outport
  wires:
  Mux1/1 -> MATLAB Function2/1(truth)
  Mux2/1 -> Scope/1, Out1/1
  Measurements from IMU/3(acc_z) -> Mux3/3
  Measurements from IMU/2(acc_y) -> Mux3/2
  Measurements from IMU/1(acc_x) -> Mux3/1
  Mux3/1 -> MATLAB Function1/1(acc_true)
  Measurements from IMU/4(vel_x) -> Mux1/1
  Measurements from IMU/5(vel_y) -> Mux1/2
  Measurements from IMU/6(vel_z) -> Mux1/3
  Mux/1 -> MATLAB Function/1(gyro_true)
  Measurements from IMU/7(wx) -> Mux/1
  Measurements from IMU/8(wy) -> Mux/2
  Measurements from IMU/9(wz) -> Mux/3
  Demux/1 -> Mux2/1
  Demux1/1 -> Mux2/2
  Demux2/2 -> Mux2/3
  MATLAB Function1/1(acc_meas) -> Demux/1
  MATLAB Function2/1(vel_meas) -> Demux1/1
  MATLAB Function/1(gyro_meas) -> Demux2/1
  MATLAB Function3/1(vel_meas) -> Demux3/1
  Acc_x1/1 -> Mux5/2
  Acc_x/1 -> Mux5/1
  Mux5/1 -> MATLAB Function3/1(truth)
  Demux3/1 -> Mux2/4
  Acc_x3/1 -> Mux6/1
  Acc_x4/1 -> Mux6/2
  Gain/1 -> Mux2/6
  FYh/1 -> MATLAB Function5/1(truth)
  Mux6/1 -> Mux2/5
  MATLAB Function5/1(vel_meas) -> Gain/1

== system generic_Truck_And_Trailer/TruckMaker/Subsystem1/Subsystem_Noisey Measurements _NAN ==
  Acc_x : TruckMaker4SL/Read CM Dict  xname=Vhcl.RL.rotv  xsync=off  xstime=Continuous
      settings: SourceProductName=TruckMaker4SL
  Acc_x1 : TruckMaker4SL/Read CM Dict  xname=Vhcl.RR.rotv  xsync=off  xstime=Continuous
      settings: SourceProductName=TruckMaker4SL
  Acc_x3 : TruckMaker4SL/Read CM Dict  xname=Tr.WheelSpd_FL  xsync=off  xstime=Continuous
      settings: SourceProductName=TruckMaker4SL
  Acc_x4 : TruckMaker4SL/Read CM Dict  xname=Tr.WheelSpd_FR  xsync=off  xstime=Continuous
      settings: SourceProductName=TruckMaker4SL
  Demux : Demux  Outputs=2
  Demux1 : Demux  Outputs=2
  Demux2 : Demux  Outputs=2
  Demux3 : Demux  Outputs=1
  FYh : TruckMaker4SL/Read CM Dict  xname=Tr.Hitch.Frc2Tr.y_1  xsync=off  xstime=Continuous
      settings: SourceProductName=TruckMaker4SL
  Gain : Gain
  MATLAB Function : MATLAB Function  TreatAsAtomicUnit=on
  MATLAB Function1 : MATLAB Function  TreatAsAtomicUnit=on
  MATLAB Function2 : MATLAB Function  TreatAsAtomicUnit=on
  MATLAB Function3 : MATLAB Function  TreatAsAtomicUnit=on
  MATLAB Function4 : MATLAB Function  TreatAsAtomicUnit=on
  Manual Switch : ManualSwitch  CurrentSetting=0
  Measurements from IMU : Subsystem  Description=Measurements from IMU Mounted in Vhcl position (3.6; 0.0;1.0)
  Mux : Mux  Inputs=3
  Mux1 : Mux  Inputs=3
  Mux2 : Mux  Inputs=6
  Mux3 : Mux  Inputs=3
  Mux4 : Mux  Inputs=2
  Mux5 : Mux  Inputs=2
  Mux6 : Mux  Inputs=2
  NaN : Constant  Value=NaN  OutDataTypeStr=Inherit: Inherit via back propagation
  Scope : Scope
      settings: ActiveDisplayYMinimum=-12.833093805155979  ActiveDisplayYMaximum=56.830382589328167  DataLoggingVariableName=ScopeData37
  Out1 : Outport
  wires:
  MATLAB Function/1(gyro_meas) -> Demux2/1
  MATLAB Function2/1(vel_meas) -> Demux1/1
  MATLAB Function1/1(acc_meas) -> Demux/1
  Demux2/2 -> Mux2/3
  Demux/1 -> Mux2/1
  Measurements from IMU/9(wz) -> Mux/3
  Measurements from IMU/8(wy) -> Mux/2
  Measurements from IMU/7(wx) -> Mux/1
  Mux/1 -> MATLAB Function/1(gyro_true)
  Measurements from IMU/6(vel_z) -> Mux1/3
  Measurements from IMU/5(vel_y) -> Mux1/2
  Measurements from IMU/4(vel_x) -> Mux1/1
  Mux3/1 -> MATLAB Function1/1(acc_true)
  Measurements from IMU/1(acc_x) -> Mux3/1
  Measurements from IMU/2(acc_y) -> Mux3/2
  Measurements from IMU/3(acc_z) -> Mux3/3
  Mux2/1 -> Scope/1, Out1/1
  Mux1/1 -> MATLAB Function2/1(truth)
  NaN/1 -> Mux4/1, Mux4/2
  Mux4/1 -> Manual Switch/2
  Demux1/1 -> Manual Switch/1
  Manual Switch/1 -> Mux2/2
  Mux5/1 -> MATLAB Function3/1(truth)
  MATLAB Function3/1(vel_meas) -> Demux3/1
  Acc_x/1 -> Mux5/1
  Acc_x1/1 -> Mux5/2
  Demux3/1 -> Mux2/4
  Acc_x3/1 -> Mux6/1
  Acc_x4/1 -> Mux6/2
  Mux6/1 -> MATLAB Function4/1(truth)
  Gain/1 -> Mux2/6
  MATLAB Function4/1(vel_meas) -> Mux2/5
  FYh/1 -> Gain/1

== system generic_Truck_And_Trailer/TruckMaker/Tractor_Subsystem /Measurements from IMU ==
  Acc_x : TruckMaker4SL/Read CM Dict  xname=Sensor.Inertial.Vhcl.VchBdy.Acc_B.x  xsync=off  xstime=Continuous
      settings: SourceProductName=TruckMaker4SL
  Acc_x1 : TruckMaker4SL/Read CM Dict  xname=Vhcl.RL.rotv  xsync=off  xstime=Continuous
      settings: SourceProductName=TruckMaker4SL
  Acc_x2 : TruckMaker4SL/Read CM Dict  xname=Vhcl.RR.rotv  xsync=off  xstime=Continuous
      settings: SourceProductName=TruckMaker4SL
  Acc_y : TruckMaker4SL/Read CM Dict  xname=Sensor.Inertial.Vhcl.VchBdy.Acc_B.y  xsync=off  xstime=Continuous
      settings: SourceProductName=TruckMaker4SL
  Omega_z : TruckMaker4SL/Read CM Dict  xname=Sensor.Inertial.Vhcl.VchBdy.Omega_B.z  xsync=off  xstime=Continuous
      settings: SourceProductName=TruckMaker4SL
  Vel_x : TruckMaker4SL/Read CM Dict  xname=Sensor.Inertial.Vhcl.VchBdy.Vel_B.x  xsync=off  xstime=Continuous
      settings: SourceProductName=TruckMaker4SL
  Vel_y : TruckMaker4SL/Read CM Dict  xname=Sensor.Inertial.Vhcl.VchBdy.Vel_B.y  xsync=off  xstime=Continuous
      settings: SourceProductName=TruckMaker4SL
  acc_x : Outport
  acc_y : Outport  Port=2
  vel_x : Outport  Port=3
  vel_y : Outport  Port=4
  wz : Outport  Port=5
  omega_rl : Outport  Port=6
  omega_rr : Outport  Port=7
  wires:
  Acc_y/1 -> acc_y/1
  Acc_x/1 -> acc_x/1
  Vel_y/1 -> vel_y/1
  Vel_x/1 -> vel_x/1
  Omega_z/1 -> wz/1
  Acc_x1/1 -> omega_rl/1
  Acc_x2/1 -> omega_rr/1
